simulink model "aero_guidance_train_2026"  (R2026a)
settings: Solver=FixedStepAuto  StopTime=20  FixedStep=0.001  AbsTol=1e-6
PreLoadFcn:
  | aero_guid_dat
StopFcn:
  | %aero_guid_plot
values from neighbouring files (symbols this model uses):
  alpha_vec = (-20:1:20)'*d2r    [aero_guid_dat.m]
  Beamwidth = 10*d2r    (= 0.174532925199)    [aero_guid_dat.m]
  Cm_alpha = am*al.^3 + bm*al.*abs(al) - cm*(7-8*M/3).*al    [aero_guid_dat.m]
  Cm_el = -0.206000/d2r    (= -11.8029305797)    [aero_guid_dat.m]
  Cm_q = -1.719    [aero_guid_dat.m]
  Cx_alpha = -0.3*ones(length(alpha_vec),length(Mach_vec))    [aero_guid_dat.m]
  Cz_alpha = an*al.^3 + bn*al.*abs(al) + cn*(2-M/3).*al    [aero_guid_dat.m]
  Cz_el = -0.034000/d2r    (= -1.94805650344)    [aero_guid_dat.m]
  d2r = pi/180    (= 0.0174532925199)    [aero_guid_dat.m]
  d_ref = 0.75/m2ft    (= 0.228599992685)    [aero_guid_dat.m]
  fin_max = 30.0*d2r    (= 0.523598775598)    [aero_guid_dat.m]
  fin_min = -30.0*d2r    (= -0.523598775598)    [aero_guid_dat.m]
  g = 9.81    [aero_guid_dat.m]
  Goal_pos = [4800; -3200]    [aero_guid_dat.m]
  h_ini = 10000/m2ft    (= 3047.99990246)    [aero_guid_dat.m]
  K_r = -0.02    [aero_guid_dat.m]
  Ks = wgyro/5    (= 125.663706144)    [aero_guid_dat.m]
  l_acc = 0.5    [aero_guid_dat.m]
  Mach_vec = 2:0.5:4    [aero_guid_dat.m]
  max_acc = 40*9.81    (= 392.4)    [aero_guid_dat.m]
  max_gimbal = 35*d2r    (= 0.610865238198)    [aero_guid_dat.m]
  min_gimbal = -35*d2r    (= -0.610865238198)    [aero_guid_dat.m]
  q_ini = 0*d2r    (= 0)    [aero_guid_dat.m]
  R_scale = 5000    [aero_guid_dat.m]
  S_ref = 0.44/m2ft^2    (= 0.0408773349839)    [aero_guid_dat.m]
  target_dt = 0.01    [aero_guid_dat.m]
  target_init_pos = pos_tgt(:)    [aero_guid_dat.m]
  target_max_turn_rate = 120 * (pi/180)    (= 2.09439510239)    [aero_guid_dat.m]
  theta_tgt = 180*d2r    (= 3.14159265359)    [aero_guid_dat.m]
  Thrust = 10e3    (= 10000)    [aero_guid_dat.m]
  tors = 0.05    [aero_guid_dat.m]
  v_ini = 3*328    (= 984)    [aero_guid_dat.m]
  V_scale = 1000    [aero_guid_dat.m]
  v_tgt = 328    [aero_guid_dat.m]
  wgyro = 100*2*pi    (= 628.318530718)    [aero_guid_dat.m]
  wn_hom = 7.0    (= 7)    [aero_guid_dat.m]
  x_ini = 0    [aero_guid_dat.m]
undefined symbols (not defined in the file or in its folder): alpha_sch, K, Ka, Kg, Ki, M_sch
libraries: aerolibasang x3, simulink x2, aerolibanim x1, aerolibatmos2 x1, aerolibactuator x1, rllib x1
CloseFcn:
  | h=findobj('type','figure');if ~isempty(h);close(h);end
Description:
  | Dynamics of a missile engaging a target which is flying straight and level
settings Model: ExtModeTrigMode=oneshot  ExtModeArmWhenConnect=off  ExtModeAutoUpdateStatusClock=off  Creator=The MathWorks, Inc.  LastModifiedBy=yunho
settings DataIOCC: StateSaveName=xbase  OutputSaveName=ybase  SignalLoggingName=sigsOut
settings OptimizationCC: InitFltsAndDblsToZero=on
settings DebuggingCC: SaveWithParameterizedLinksMsg=none  SignalResolutionControl=TryResolveAllWithWarning  MultiTaskDSMMsg=warning  MultiTaskCondExecSysMsg=none  SigSpecEnsureSampleTimeMsg=none
settings HardwareCC: ProdHWDeviceType=32-bit Generic
settings GRTTargetCC: TargetFcnLib=ansi_tfl_tmw.mat  CombineOutputUpdateFcns=off  GRTInterface=on
settings ConfigComp: CovMetricSettings=d

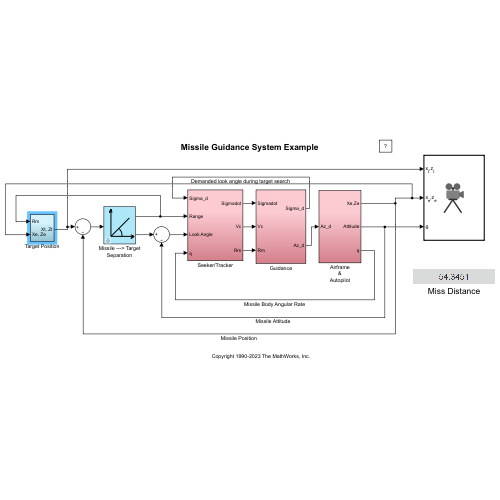
[thumbnail: Simulink's stored preview of the top-level diagram]
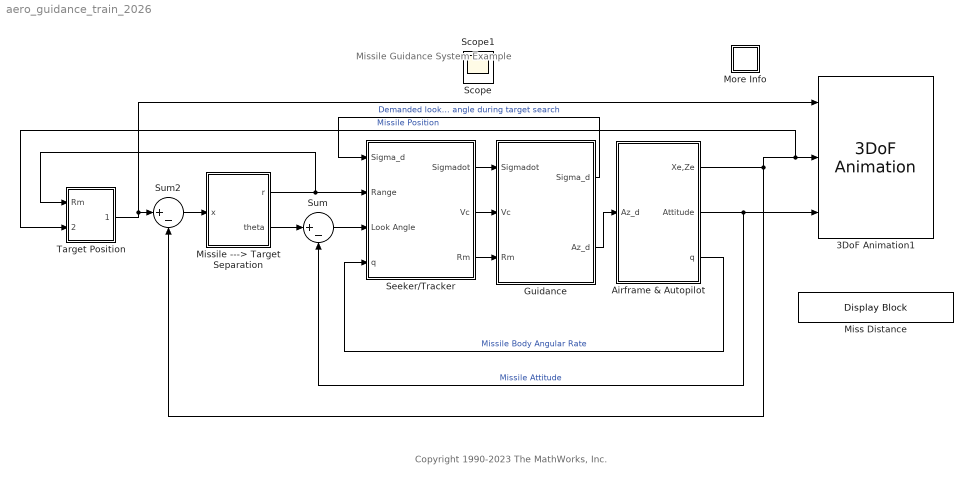
== system aero_guidance_train_2026 ==
  note: Copyright 1990-2023 The MathWorks, Inc.
  note: Missile Guidance System Example
  3DoF Animation1 : aerolibanim/3DoF Animation  u1=[0 5000 -2000 2000 -5050 -3050]  u2=0.01  u3=4  u5=Fixed position  u6=[2500 4000 -4050]  u7=40  u8=on
  Airframe & Autopilot : Subsystem
  Guidance : Subsystem
  Miss Distance : DisplayBlock  LabelPosition=Hide  Transparency=1  GridColor=[0.0, 0.0, 0.0]
  Missile ---> Target Separation : Subsystem  mask(Cart2Polar){}
      mask help:
      | Transformation from cartesian to polar coordinates.
      | [x, y] -> [r, theta]
      |
      | r = sqrt(x^2 + y^2);
      | theta = atan(y/x);
      mask Help: Unmask this block for more help.
      mask Display: plot(0,0,100,100,[24,20,15,20,20],[85,95,85,95,20],[80,20,95,85,95,85],[70,20,20,15,20,24],[56,56,55,52,50,46],[20,26,31,35,38,42])
  More Info : Subsystem
      settings: OpenFcn=showExample('simulink_aerospace/DesigningAGuidanceSystemInMATLABAndSimulinkExample')
      mask Display: disp('?')
  Seeker/Tracker : Subsystem
  Sum : Sum  Inputs=|+-  InputSameDT=on  SaturateOnIntegerOverflow=on  OutDataTypeStr=Inherit: Same as first input
  Sum2 : Sum  Inputs=|+-  InputSameDT=on  SaturateOnIntegerOverflow=on  OutDataTypeStr=Inherit: Same as first input
  Target Position : Subsystem
  Scope : Scope
  Scope1 : Scope
  wires:
  Missile ---> Target Separation/2(theta) -> Sum/1
  Guidance/2(Az_d) -> Airframe & Autopilot/1(Az_d)
  Seeker/Tracker/2(Vc) -> Guidance/2(Vc)
  Seeker/Tracker/3(Rm) -> Guidance/3(Rm)
  Seeker/Tracker/1(Sigmadot) -> Guidance/1(Sigmadot)
  Sum/1 -> Seeker/Tracker/3(Look Angle)
  Airframe & Autopilot/3(q) -> Seeker/Tracker/4(q)  "Missile Body Angular Rate"
  Guidance/1(Sigma_d) -> Seeker/Tracker/1(Sigma_d)  "Demanded look angle during target search"
  Missile ---> Target Separation/1(r) -> Target Position/1(Rm), Seeker/Tracker/2(Range)
  Airframe & Autopilot/1(Xe,Ze) -> Target Position/2("Xe, Ze"), 3DoF Animation1/2, Sum2/2  "Missile Position"
  Airframe & Autopilot/2(Attitude) -> Sum/2, 3DoF Animation1/3  "Missile Attitude"
  Sum2/1 -> Missile ---> Target Separation/1(x)
  Target Position/1("Xt, Zt") -> 3DoF Animation1/1, Sum2/1

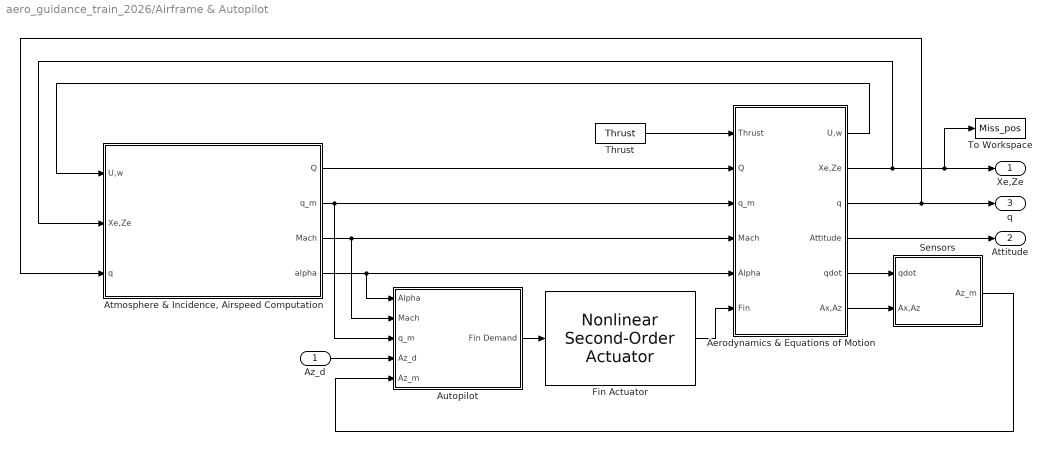
== system aero_guidance_train_2026/Airframe & Autopilot ==
  Az_d : Inport
  Aerodynamics & Equations of Motion : Subsystem
  "Atmosphere & Incidence, Airspeed Computation" : Subsystem
  Autopilot : Subsystem
  Fin Actuator : aerolibactuator/Nonlinear Second-Order Actuator  wn_fin=wn_fin  z_fin=z_fin  fin_max=fin_max  fin_min=fin_min  fin_maxrate=fin_maxrate  fin_act_0=fin_act_0  fin_act_vel=0
  Sensors : Subsystem
  Thrust : Constant  Value=Thrust
  To Workspace : ToWorkspace  VariableName=Miss_pos  SaveFormat=Structure With Time  SampleTime=-1
  Xe,Ze : Outport  InitialOutput=0  VectorParamsAs1DForOutWhenUnconnected=off
  Attitude : Outport  Port=2  InitialOutput=0  VectorParamsAs1DForOutWhenUnconnected=off
  q : Outport  Port=3  InitialOutput=0  VectorParamsAs1DForOutWhenUnconnected=off
  wires:
  Thrust/1 -> Aerodynamics & Equations of Motion/1(Thrust)
  Aerodynamics & Equations of Motion/3(q) -> q/1, "Atmosphere & Incidence, Airspeed Computation"/3(q)
  Aerodynamics & Equations of Motion/2(Xe,Ze) -> To Workspace/1, Xe,Ze/1, "Atmosphere & Incidence, Airspeed Computation"/2(Xe,Ze)
  "Atmosphere & Incidence, Airspeed Computation"/3(Mach) -> Aerodynamics & Equations of Motion/4(Mach), Autopilot/2(Mach)
  Aerodynamics & Equations of Motion/1(U,w) -> "Atmosphere & Incidence, Airspeed Computation"/1(U,w)
  "Atmosphere & Incidence, Airspeed Computation"/1(Q) -> Aerodynamics & Equations of Motion/2(Q)
  "Atmosphere & Incidence, Airspeed Computation"/4(alpha) -> Autopilot/1(Alpha), Aerodynamics & Equations of Motion/5(Alpha)
  "Atmosphere & Incidence, Airspeed Computation"/2(q_m) -> Aerodynamics & Equations of Motion/3(q_m), Autopilot/3(q_m)
  Aerodynamics & Equations of Motion/4(Attitude) -> Attitude/1
  Aerodynamics & Equations of Motion/5(qdot) -> Sensors/1(qdot)
  Aerodynamics & Equations of Motion/6(Ax,Az) -> Sensors/2(Ax,Az)
  Autopilot/1(Fin Demand) -> Fin Actuator/1
  Fin Actuator/1 -> Aerodynamics & Equations of Motion/6(Fin)
  Az_d/1 -> Autopilot/4(Az_d)
  Sensors/1(Az_m) -> Autopilot/5(Az_m)

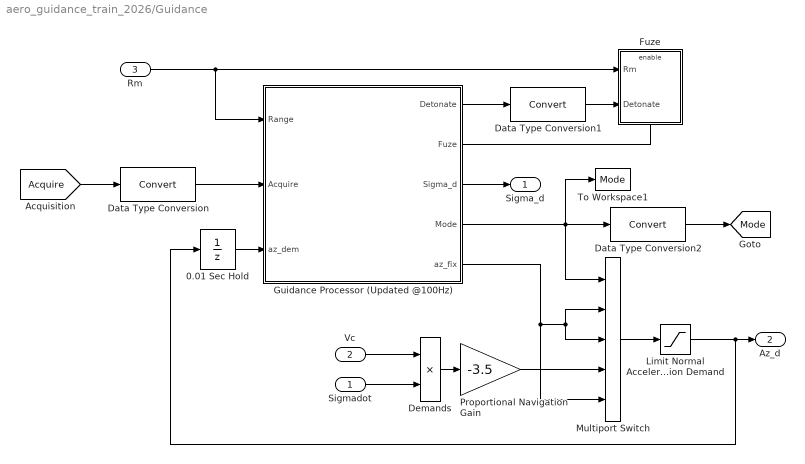
== system aero_guidance_train_2026/Guidance ==
  Sigmadot : Inport
  Vc : Inport  Port=2
  Rm : Inport  Port=3
  0.01 Sec Hold : UnitDelay  SampleTime=0.01
  Data Type Conversion : DataTypeConversion  SaturateOnIntegerOverflow=off  RndMeth=Floor
  Data Type Conversion1 : DataTypeConversion  SaturateOnIntegerOverflow=off  RndMeth=Floor
  Data Type Conversion2 : DataTypeConversion  SaturateOnIntegerOverflow=off  RndMeth=Floor
  Demands : Product  InputSameDT=on  SaturateOnIntegerOverflow=on  OutDataTypeStr=Inherit: Same as first input
  Fuze : Subsystem  TreatAsAtomicUnit=on
  Guidance Processor (Updated @100Hz) : Stateflow chart  TreatAsAtomicUnit=on
  "Limit Normal Acceleration Demand " : Saturate  UpperLimit=max_acc  LowerLimit=-max_acc
  Multiport Switch : MultiPortSwitch  Inputs=4
  Proportional Navigation Gain : Gain  Gain=-3.5  SaturateOnIntegerOverflow=on  OutDataTypeStr=Inherit: Same as input  ParamDataTypeStr=Inherit: Same as input
  To Workspace1 : ToWorkspace  VariableName=Mode  SaveFormat=Structure With Time
  Sigma_d : Outport  VectorParamsAs1DForOutWhenUnconnected=off
  Az_d : Outport  Port=2  VectorParamsAs1DForOutWhenUnconnected=off
  tag scope: Mode=global
  wires:
  Guidance Processor (Updated @100Hz)/3(Sigma_d) -> Sigma_d/1
  [Acquire] -> Data Type Conversion/1
  Multiport Switch/1 -> "Limit Normal Acceleration Demand "/1
  Guidance Processor (Updated @100Hz)/1(Detonate) -> Data Type Conversion1/1
  "Limit Normal Acceleration Demand "/1 -> Az_d/1, 0.01 Sec Hold/1
  Guidance Processor (Updated @100Hz)/5(az_fix) -> Multiport Switch/2, Multiport Switch/3, Multiport Switch/5
  0.01 Sec Hold/1 -> Guidance Processor (Updated @100Hz)/3(az_dem)
  Sigmadot/1 -> Demands/2
  Proportional Navigation Gain/1 -> Multiport Switch/4
  Vc/1 -> Demands/1
  Demands/1 -> Proportional Navigation Gain/1
  Rm/1 -> Fuze/1(Rm), Guidance Processor (Updated @100Hz)/1(Range)
  Guidance Processor (Updated @100Hz)/2(Fuze) -> Fuze/Enable
  Guidance Processor (Updated @100Hz)/4(Mode) -> Data Type Conversion2/1, To Workspace1/1, Multiport Switch/1
  Data Type Conversion/1 -> Guidance Processor (Updated @100Hz)/2(Acquire)
  Data Type Conversion1/1 -> Fuze/2(Detonate)
  Data Type Conversion2/1 -> [Mode]

== system aero_guidance_train_2026/Missile ---> Target Separation ==
  x : Inport
  Range : Fcn  Expr=hypot(u[1],u[2])
  Sightline Angle : Fcn  Expr=atan2(-u[2],u[1])
  r : Outport  InitialOutput=0  VectorParamsAs1DForOutWhenUnconnected=off
  theta : Outport  Port=2  InitialOutput=0  VectorParamsAs1DForOutWhenUnconnected=off
  wires:
  x/1 -> Sightline Angle/1, Range/1
  Range/1 -> r/1
  Sightline Angle/1 -> theta/1

== system aero_guidance_train_2026/More Info ==

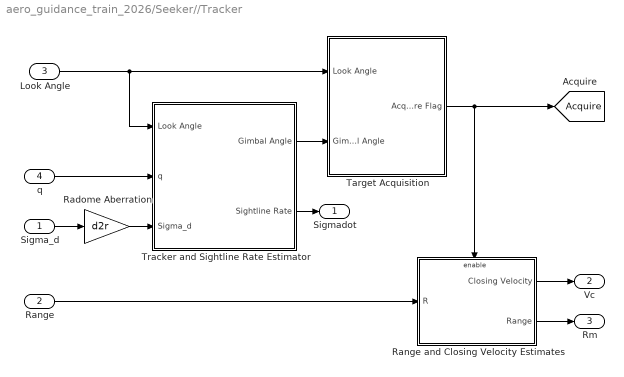
== system aero_guidance_train_2026/Seeker//Tracker ==
  Sigma_d : Inport
  Range : Inport  Port=2
  Look Angle : Inport  Port=3
  q : Inport  Port=4
  Radome Aberration : Gain  Gain=d2r  SaturateOnIntegerOverflow=on  OutDataTypeStr=Inherit: Same as input  ParamDataTypeStr=Inherit: Same as input
  Range and Closing Velocity Estimates : Subsystem  TreatAsAtomicUnit=on
  Target Acquisition : Subsystem
  Tracker and Sightline Rate Estimator : Subsystem
  Sigmadot : Outport  VectorParamsAs1DForOutWhenUnconnected=off
  Vc : Outport  Port=2  VectorParamsAs1DForOutWhenUnconnected=off
  Rm : Outport  Port=3  VectorParamsAs1DForOutWhenUnconnected=off
  tag scope: Acquire=global
  wires:
  Tracker and Sightline Rate Estimator/2(Sightline Rate) -> Sigmadot/1
  Radome Aberration/1 -> Tracker and Sightline Rate Estimator/3(Sigma_d)
  Tracker and Sightline Rate Estimator/1("Gimbal Angle ") -> Target Acquisition/2(Gimbal Angle)
  Target Acquisition/1(Acquire Flag) -> [Acquire], Range and Closing Velocity Estimates/Enable
  q/1 -> Tracker and Sightline Rate Estimator/2(q)
  Look Angle/1 -> Target Acquisition/1(Look Angle), Tracker and Sightline Rate Estimator/1(Look Angle)
  Range/1 -> Range and Closing Velocity Estimates/1(R)
  Range and Closing Velocity Estimates/2(Range) -> Rm/1
  Range and Closing Velocity Estimates/1(Closing Velocity) -> Vc/1
  Sigma_d/1 -> Radome Aberration/1

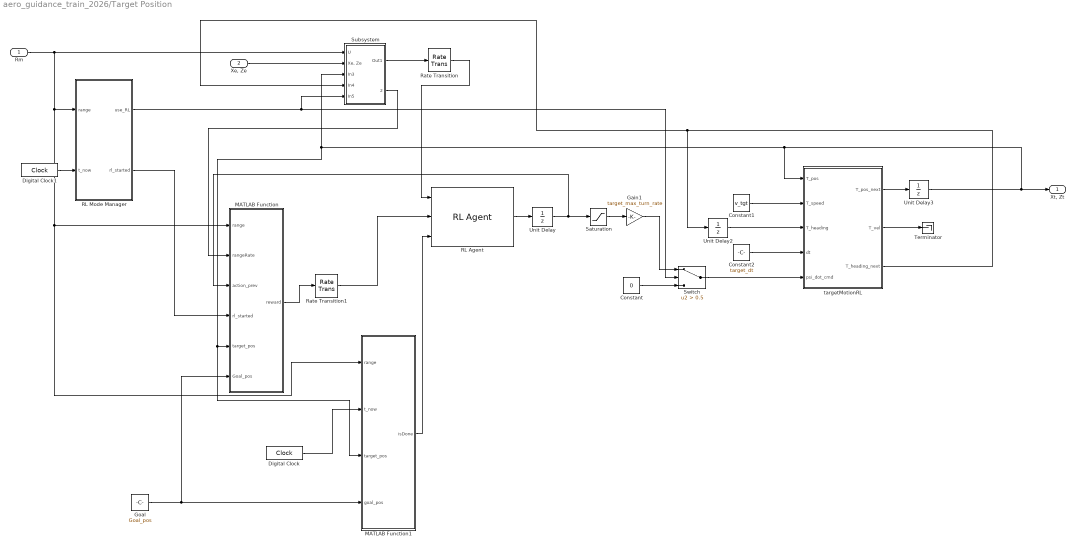
== system aero_guidance_train_2026/Target Position ==
  Rm : Inport
  "Xe, Ze" : Inport  Port=2
  Constant : Constant  Value=0
  Constant1 : Constant  Value=v_tgt
  Constant2 : Constant  Value=target_dt
  Digital Clock : DigitalClock  SampleTime=target_dt
  Digital Clock1 : DigitalClock  SampleTime=target_dt
  Gain1 : Gain  Gain=target_max_turn_rate
  Goal : Constant  Value=Goal_pos  SampleTime=target_dt
  MATLAB Function : MATLAB Function  TreatAsAtomicUnit=on
  MATLAB Function1 : MATLAB Function  TreatAsAtomicUnit=on
  RL Agent : rllib/RL Agent  Agent=agent  ExternalActionAsInput=off  ProvideLastAction=off  ProvideCumRwd=off  TreatAsDirectFeedthrough=on  UseStrictObservationDataTypes=off
  RL Mode Manager : MATLAB Function  TreatAsAtomicUnit=on  SystemSampleTime=target_dt
  Rate Transition : RateTransition  OutPortSampleTime=target_dt
  Rate Transition1 : RateTransition  OutPortSampleTime=target_dt
  Saturation : Saturate  UpperLimit=1  LowerLimit=-1
  Subsystem : Subsystem
  Switch : Switch  Criteria=u2 > Threshold  Threshold=0.5  SaturateOnIntegerOverflow=off  InputSameDT=off
  Terminator : Terminator
  Unit Delay : UnitDelay  SampleTime=0.01
  Unit Delay2 : UnitDelay  InitialCondition=theta_tgt  SampleTime=target_dt
  Unit Delay3 : UnitDelay  InitialCondition=target_init_pos  SampleTime=target_dt
  targetMotionRL : MATLAB Function  TreatAsAtomicUnit=on  SystemSampleTime=target_dt
  "Xt, Zt" : Outport
  wires:
  RL Agent/1 -> Unit Delay/1
  Saturation/1 -> Gain1/1
  Gain1/1 -> Switch/1
  RL Mode Manager/1(use_RL) -> Subsystem/5(In5), Switch/2
  Constant/1 -> Switch/3
  Switch/1 -> targetMotionRL/5(psi_dot_cmd)
  Rm/1 -> MATLAB Function1/1(range), MATLAB Function/1(range), RL Mode Manager/1(range), Subsystem/1(U)
  "Xe, Ze"/1 -> Subsystem/2("Xe, Ze")
  targetMotionRL/1(T_pos_next) -> Unit Delay3/1
  targetMotionRL/3(T_heading_next) -> Subsystem/4(In4), Unit Delay2/1
  Subsystem/2(rangeRate_raw) -> MATLAB Function/2(rangeRate)
  Unit Delay/1 -> Saturation/1, MATLAB Function/3(action_prev)
  RL Mode Manager/2(rl_started) -> MATLAB Function/4(rl_started)
  Digital Clock/1 -> MATLAB Function1/2(t_now)
  Constant1/1 -> targetMotionRL/2(T_speed)
  Unit Delay2/1 -> targetMotionRL/3(T_heading)
  Constant2/1 -> targetMotionRL/4(dt)
  targetMotionRL/2(T_vel) -> Terminator/1
  Subsystem/1(Out1) -> Rate Transition/1
  Rate Transition/1 -> RL Agent/1
  MATLAB Function/1(reward) -> Rate Transition1/1
  Rate Transition1/1 -> RL Agent/2
  Unit Delay3/1 -> targetMotionRL/1(T_pos), MATLAB Function1/3(target_pos), MATLAB Function/5(target_pos), Subsystem/3(In3), "Xt, Zt"/1
  Digital Clock1/1 -> RL Mode Manager/2(t_now)
  MATLAB Function1/1(isDone) -> RL Agent/3
  Goal/1 -> MATLAB Function/6(Goal_pos), MATLAB Function1/4(goal_pos)

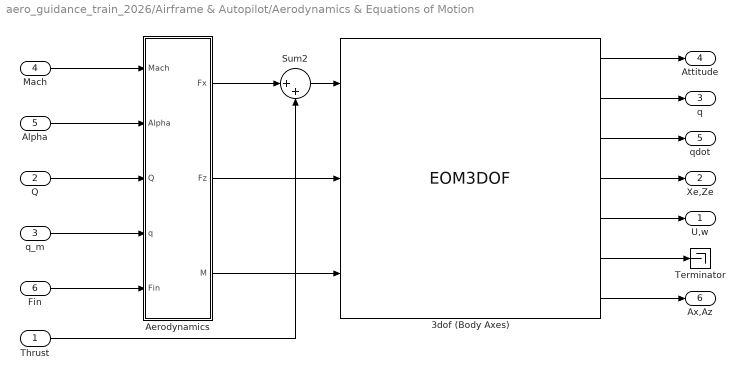
== system aero_guidance_train_2026/Airframe & Autopilot/Aerodynamics & Equations of Motion ==
  Thrust : Inport
  Q : Inport  Port=2
  q_m : Inport  Port=3
  Mach : Inport  Port=4
  Alpha : Inport  Port=5
  Fin : Inport  Port=6
  3dof (Body Axes) : EOM3DOF  v_ini=v_ini  theta_ini=theta_ini  q_ini=q_ini  alpha_ini=alpha_ini  pos_ini=[x_ini -h_ini]  mass=mass  Iyy=Iyy  g=g  abi_flag=on
  Aerodynamics : Subsystem
  Sum2 : Sum  Inputs=|++  InputSameDT=on  SaturateOnIntegerOverflow=on  OutDataTypeStr=Inherit: Same as first input
  Terminator : Terminator
  U,w : Outport  InitialOutput=0  VectorParamsAs1DForOutWhenUnconnected=off
  Xe,Ze : Outport  Port=2  InitialOutput=0  VectorParamsAs1DForOutWhenUnconnected=off
  q : Outport  Port=3  InitialOutput=0  VectorParamsAs1DForOutWhenUnconnected=off
  Attitude : Outport  Port=4  InitialOutput=0  VectorParamsAs1DForOutWhenUnconnected=off
  qdot : Outport  Port=5  InitialOutput=0  VectorParamsAs1DForOutWhenUnconnected=off
  Ax,Az : Outport  Port=6  InitialOutput=0  VectorParamsAs1DForOutWhenUnconnected=off
  wires:
  Aerodynamics/3(" M") -> 3dof (Body Axes)/3
  Sum2/1 -> 3dof (Body Axes)/1
  Fin/1 -> Aerodynamics/5(Fin)
  Aerodynamics/2(Fz) -> 3dof (Body Axes)/2
  Aerodynamics/1(Fx) -> Sum2/1
  Thrust/1 -> Sum2/2
  q_m/1 -> Aerodynamics/4(q)
  Mach/1 -> Aerodynamics/1(Mach)
  Q/1 -> Aerodynamics/3(Q)
  Alpha/1 -> Aerodynamics/2(Alpha)
  3dof (Body Axes)/7 -> Ax,Az/1
  3dof (Body Axes)/6 -> Terminator/1
  3dof (Body Axes)/5 -> U,w/1
  3dof (Body Axes)/4 -> Xe,Ze/1
  3dof (Body Axes)/3 -> qdot/1
  3dof (Body Axes)/2 -> q/1
  3dof (Body Axes)/1 -> Attitude/1

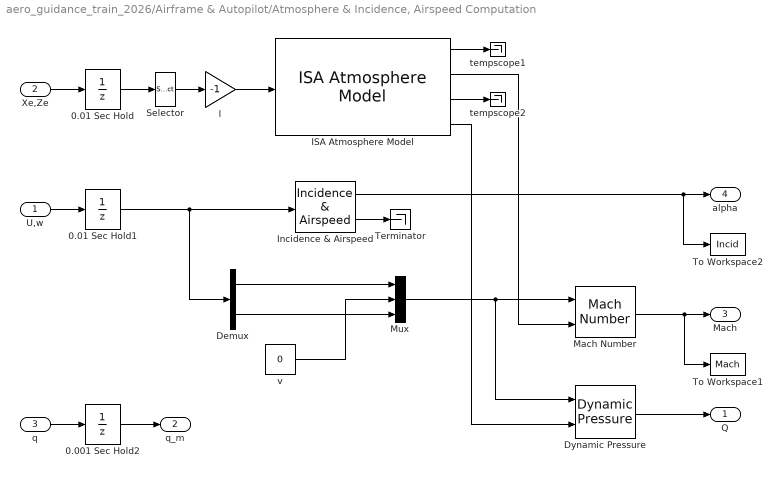
== system aero_guidance_train_2026/Airframe & Autopilot/Atmosphere & Incidence, Airspeed Computation ==
  U,w : Inport
  Xe,Ze : Inport  Port=2
  q : Inport  Port=3
  0.001 Sec Hold2 : UnitDelay  InitialCondition=q_ini  SampleTime=0.001
  0.01 Sec Hold : UnitDelay  InitialCondition=[x_ini -h_ini]  SampleTime=0.01
  0.01 Sec Hold1 : UnitDelay  InitialCondition=[v_ini 0]  SampleTime=0.01
  Demux : Demux  Outputs=2
  Dynamic Pressure : aerolibasang/Dynamic Pressure
  ISA Atmosphere Model : aerolibatmos2/ISA Atmosphere Model  useExtended=off  action=Warning  custom=off  viscosityOut=off  g=9.80665  gamma=1.4  R=287.0531  L=0.0065  h_trop=11000  h_strat=20000  rho0=1.225  P0=101325  T0=288.15  h0=0  S=110.4  Tref=273.15  muref=1.716e-5
  Incidence & Airspeed : aerolibasang/Incidence  & Airspeed
  Mach Number : aerolibasang/Mach Number
  Mux : Mux  Inputs=3
  Selector : Selector  InputPortWidth=2  IndexOptions=Index vector (dialog)  Indices=[2]  OutputSizes=1
  Terminator : Terminator
  To Workspace1 : ToWorkspace  VariableName=Mach  SaveFormat=Structure With Time  SampleTime=-1
  To Workspace2 : ToWorkspace  VariableName=Incid  SaveFormat=Structure With Time  SampleTime=-1
  l : Gain  Gain=-1  SaturateOnIntegerOverflow=on  OutDataTypeStr=Inherit: Same as input  ParamDataTypeStr=Inherit: Same as input
  tempscope1 : Terminator
  tempscope2 : Terminator
  v : Constant  Value=0
  Q : Outport
  q_m : Outport  Port=2
  Mach : Outport  Port=3
  alpha : Outport  Port=4
  wires:
  U,w/1 -> 0.01 Sec Hold1/1
  Incidence & Airspeed/1 -> To Workspace2/1, alpha/1
  Demux/1 -> Mux/1
  Demux/2 -> Mux/3
  v/1 -> Mux/2
  Mux/1 -> Mach Number/1, Dynamic Pressure/1
  Incidence & Airspeed/2 -> Terminator/1
  ISA Atmosphere Model/4 -> Dynamic Pressure/2
  Mach Number/1 -> To Workspace1/1, Mach/1
  Dynamic Pressure/1 -> Q/1
  0.01 Sec Hold1/1 -> Incidence & Airspeed/1, Demux/1
  0.01 Sec Hold/1 -> Selector/1
  l/1 -> ISA Atmosphere Model/1
  ISA Atmosphere Model/1 -> tempscope1/1
  ISA Atmosphere Model/3 -> tempscope2/1
  Selector/1 -> l/1
  Xe,Ze/1 -> 0.01 Sec Hold/1
  ISA Atmosphere Model/2 -> Mach Number/2
  0.001 Sec Hold2/1 -> q_m/1
  q/1 -> 0.001 Sec Hold2/1

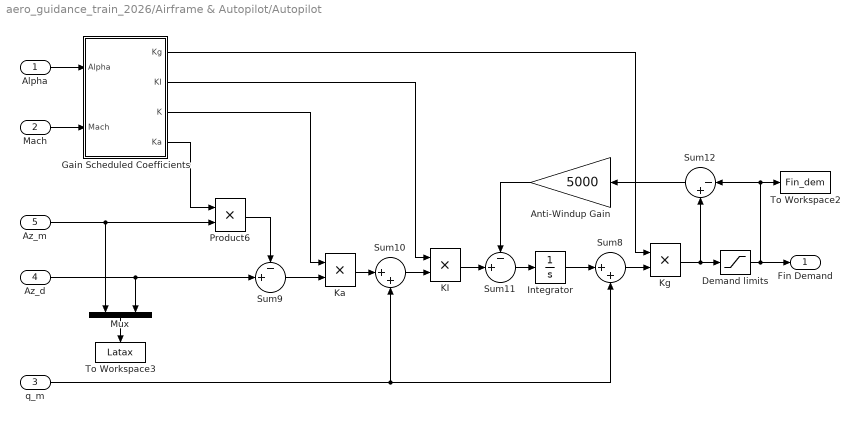
== system aero_guidance_train_2026/Airframe & Autopilot/Autopilot ==
  Alpha : Inport
  Mach : Inport  Port=2
  q_m : Inport  Port=3
  Az_d : Inport  Port=4
  Az_m : Inport  Port=5
  Anti-Windup Gain : Gain  Gain=5000  SaturateOnIntegerOverflow=on  OutDataTypeStr=Inherit: Same as input  ParamDataTypeStr=Inherit: Same as input
  "Demand limits " : Saturate  UpperLimit=fin_max  LowerLimit=fin_min
  Gain Scheduled Coefficients : Subsystem
  Integrator : Integrator
  KI : Product  InputSameDT=on  SaturateOnIntegerOverflow=on  OutDataTypeStr=Inherit: Same as first input
  Ka : Product  InputSameDT=on  SaturateOnIntegerOverflow=on  OutDataTypeStr=Inherit: Same as first input
  Kg : Product  InputSameDT=on  SaturateOnIntegerOverflow=on  OutDataTypeStr=Inherit: Same as first input
  Mux : Mux  Inputs=2
  Product6 : Product  InputSameDT=on  SaturateOnIntegerOverflow=on  OutDataTypeStr=Inherit: Same as first input
  Sum10 : Sum  Inputs=|++  InputSameDT=on  SaturateOnIntegerOverflow=on  OutDataTypeStr=Inherit: Same as first input
  Sum11 : Sum  Inputs=-+|  InputSameDT=on  SaturateOnIntegerOverflow=on  OutDataTypeStr=Inherit: Same as first input
  Sum12 : Sum  Inputs=|-+  InputSameDT=on  SaturateOnIntegerOverflow=on  OutDataTypeStr=Inherit: Same as first input
  Sum8 : Sum  Inputs=|++  InputSameDT=on  SaturateOnIntegerOverflow=on  OutDataTypeStr=Inherit: Same as first input
  Sum9 : Sum  Inputs=-+|  InputSameDT=on  SaturateOnIntegerOverflow=on  OutDataTypeStr=Inherit: Same as first input
  To Workspace2 : ToWorkspace  VariableName=Fin_dem  SaveFormat=Structure With Time  SampleTime=-1
  To Workspace3 : ToWorkspace  VariableName=Latax  SaveFormat=Structure With Time  SampleTime=-1
  Fin Demand : Outport  InitialOutput=0  VectorParamsAs1DForOutWhenUnconnected=off
  wires:
  Mach/1 -> Gain Scheduled Coefficients/2(Mach)
  Alpha/1 -> Gain Scheduled Coefficients/1(Alpha)
  Kg/1 -> Sum12/2, "Demand limits "/1
  Gain Scheduled Coefficients/1("Kg ") -> Kg/1
  Gain Scheduled Coefficients/3("K ") -> Ka/1
  Gain Scheduled Coefficients/2("KI ") -> KI/1
  Anti-Windup Gain/1 -> Sum11/1
  Sum8/1 -> Kg/2
  Integrator/1 -> Sum8/1
  Sum11/1 -> Integrator/1
  Product6/1 -> Sum9/1
  Sum9/1 -> Ka/2
  Ka/1 -> Sum10/1
  Sum10/1 -> KI/2
  KI/1 -> Sum11/2
  Sum12/1 -> Anti-Windup Gain/1
  Az_d/1 -> Mux/2, Sum9/2
  Mux/1 -> To Workspace3/1
  q_m/1 -> Sum10/2, Sum8/2
  "Demand limits "/1 -> Fin Demand/1, Sum12/1, To Workspace2/1
  Az_m/1 -> Mux/1, Product6/2
  Gain Scheduled Coefficients/4("Ka ") -> Product6/1

== system aero_guidance_train_2026/Airframe & Autopilot/Sensors ==
  qdot : Inport
  Ax,Az : Inport  Port=2
  Selector : Selector  InputPortWidth=2  IndexOptions=Index vector (dialog)  Indices=[2]  OutputSizes=1
  Sum : Sum  Inputs=-+|  InputSameDT=on  SaturateOnIntegerOverflow=on  OutDataTypeStr=Inherit: Same as first input
  l : Gain  Gain=l_acc  SaturateOnIntegerOverflow=on  OutDataTypeStr=Inherit: Same as input  ParamDataTypeStr=Inherit: Same as input
  Az_m : Outport  InitialOutput=0  VectorParamsAs1DForOutWhenUnconnected=off
  wires:
  Selector/1 -> Sum/2
  Ax,Az/1 -> Selector/1
  l/1 -> Sum/1
  Sum/1 -> Az_m/1  "Accelerometer"
  qdot/1 -> l/1

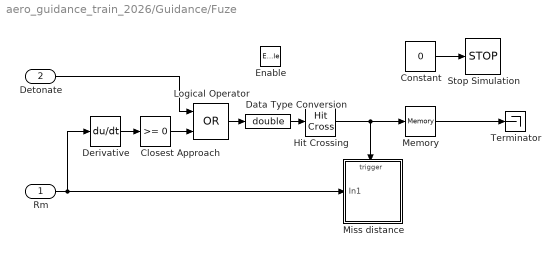
== system aero_guidance_train_2026/Guidance/Fuze ==
  Rm : Inport
  Detonate : Inport  Port=2
  Enable : EnablePort
  Closest Approach : simulink/Logic and Bit Operations/Compare To Zero  relop=>=  OutDataTypeStr=boolean
  Constant : Constant  Value=0
  Data Type Conversion : DataTypeConversion  OutDataTypeStr=double  SaturateOnIntegerOverflow=off  RndMeth=Floor
  Derivative : Derivative
  Hit Crossing : HitCross  HitCrossingDirection=rising
  Logical Operator : Logic  Operator=OR  IconShape=distinctive  OutDataTypeStr=boolean
  Memory : Memory
  Miss distance : Subsystem  TreatAsAtomicUnit=on
  Stop Simulation : Stop
  Terminator : Terminator
  wires:
  Derivative/1 -> Closest Approach/1
  Detonate/1 -> Logical Operator/1
  Rm/1 -> Miss distance/1(In1), Derivative/1
  Closest Approach/1 -> Logical Operator/2
  Memory/1 -> Terminator/1
  Hit Crossing/1 -> Miss distance/Trigger, Memory/1
  Data Type Conversion/1 -> Hit Crossing/1
  Logical Operator/1 -> Data Type Conversion/1
  Constant/1 -> Stop Simulation/1

== system aero_guidance_train_2026/Seeker//Tracker/Range and Closing Velocity Estimates ==
  R : Inport
  Enable : EnablePort  StatesWhenEnabling=reset
  Bandwidth of Estimator : Gain  Gain=wn_hom  SaturateOnIntegerOverflow=on  OutDataTypeStr=Inherit: Same as input  ParamDataTypeStr=Inherit: Same as input
  Initialized at acquisition : Integrator  InitialConditionSource=external
  Rdot ---> Vc : Gain  Gain=-1  SaturateOnIntegerOverflow=on  OutDataTypeStr=Inherit: Same as input  ParamDataTypeStr=Inherit: Same as input
  Sum : Sum  Inputs=|+-  InputSameDT=on  SaturateOnIntegerOverflow=on  OutDataTypeStr=Inherit: Same as first input
  Closing Velocity : Outport  InitialOutput=0  VectorParamsAs1DForOutWhenUnconnected=off
  Range : Outport  Port=2  InitialOutput=0  VectorParamsAs1DForOutWhenUnconnected=off
  wires:
  R/1 -> Range/1, Initialized at acquisition/2, Sum/1
  Sum/1 -> Bandwidth of Estimator/1
  Initialized at acquisition/1 -> Sum/2
  Bandwidth of Estimator/1 -> Rdot ---> Vc/1, Initialized at acquisition/1
  Rdot ---> Vc/1 -> Closing Velocity/1

== system aero_guidance_train_2026/Seeker//Tracker/Target Acquisition ==
  Look Angle : Inport
  Gimbal Angle : Inport  Port=2
  Abs : Abs
  Beamwidth : Constant  Value=Beamwidth/2
  Mux : Mux  Inputs=2
  Relational Operator : RelationalOperator  Operator=<  OutDataTypeStr=boolean
  Sum : Sum  Inputs=+-  InputSameDT=on  SaturateOnIntegerOverflow=on  OutDataTypeStr=Inherit: Same as first input
  To Workspace2 : ToWorkspace  VariableName=Gimbal  SaveFormat=Structure With Time  SampleTime=-1
  Acquire Flag : Outport  VectorParamsAs1DForOutWhenUnconnected=off
  wires:
  Look Angle/1 -> Sum/2, Mux/2
  Gimbal Angle/1 -> Sum/1, Mux/1
  Mux/1 -> To Workspace2/1
  Sum/1 -> Abs/1
  Beamwidth/1 -> Relational Operator/2
  Relational Operator/1 -> Acquire Flag/1
  Abs/1 -> Relational Operator/1

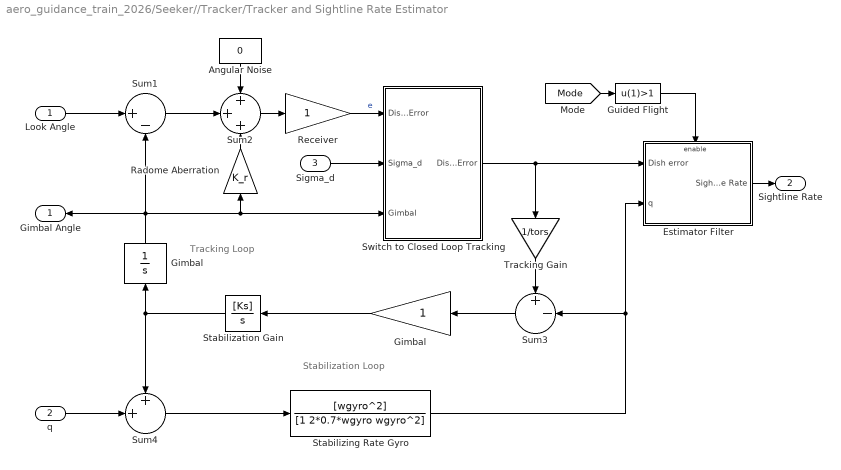
== system aero_guidance_train_2026/Seeker//Tracker/Tracker and Sightline Rate Estimator ==
  note: Stabilization Loop
  note: Tracking Loop
  Look Angle : Inport
  q : Inport  Port=2
  Sigma_d : Inport  Port=3
  Angular Noise : Constant  Value=0
  Estimator Filter : Subsystem  TreatAsAtomicUnit=on
  Gimbal : Gain  SaturateOnIntegerOverflow=on  OutDataTypeStr=Inherit: Same as input  ParamDataTypeStr=Inherit: Same as input
  "Gimbal " : Integrator  LimitOutput=on  UpperSaturationLimit=max_gimbal  LowerSaturationLimit=min_gimbal
  Guided Flight : Fcn  Expr=u(1)>1
  Radome Aberration : Gain  Gain=K_r  SaturateOnIntegerOverflow=on  OutDataTypeStr=Inherit: Same as input  ParamDataTypeStr=Inherit: Same as input
  Receiver : Gain  SaturateOnIntegerOverflow=on  OutDataTypeStr=Inherit: Same as input  ParamDataTypeStr=Inherit: Same as input
  Stabilization Gain : TransferFcn  Numerator=[Ks]  Denominator=[1 0]
  Stabilizing Rate Gyro : TransferFcn  Numerator=[wgyro^2]  Denominator=[1 2*0.7*wgyro wgyro^2]
  Sum1 : Sum  Inputs=|+-  InputSameDT=on  SaturateOnIntegerOverflow=on  OutDataTypeStr=Inherit: Same as first input
  Sum2 : Sum  Inputs=+++  InputSameDT=on  SaturateOnIntegerOverflow=on  OutDataTypeStr=Inherit: Same as first input
  Sum3 : Sum  Inputs=+-|  InputSameDT=on  SaturateOnIntegerOverflow=on  OutDataTypeStr=Inherit: Same as first input
  Sum4 : Sum  Inputs=++|  InputSameDT=on  SaturateOnIntegerOverflow=on  OutDataTypeStr=Inherit: Same as first input
  Switch to Closed Loop Tracking : Subsystem
  Tracking Gain : Gain  Gain=1/tors  SaturateOnIntegerOverflow=on  OutDataTypeStr=Inherit: Same as input  ParamDataTypeStr=Inherit: Same as input
  "Gimbal Angle " : Outport  VectorParamsAs1DForOutWhenUnconnected=off
  Sightline Rate : Outport  Port=2  VectorParamsAs1DForOutWhenUnconnected=off
  wires:
  "Gimbal "/1 -> Sum1/2, Radome Aberration/1, Switch to Closed Loop Tracking/3(Gimbal), "Gimbal Angle "/1
  Stabilization Gain/1 -> "Gimbal "/1, Sum4/1
  Gimbal/1 -> Stabilization Gain/1
  Look Angle/1 -> Sum1/1
  Sum2/1 -> Receiver/1
  Receiver/1 -> Switch to Closed Loop Tracking/1(Dish Error)  "e"
  Sigma_d/1 -> Switch to Closed Loop Tracking/2(Sigma_d)
  Estimator Filter/1(Sightline Rate) -> Sightline Rate/1
  Radome Aberration/1 -> Sum2/3
  Sum1/1 -> Sum2/2
  Angular Noise/1 -> Sum2/1
  Sum4/1 -> Stabilizing Rate Gyro/1
  q/1 -> Sum4/2
  Stabilizing Rate Gyro/1 -> Sum3/2, Estimator Filter/2(q)
  Sum3/1 -> Gimbal/1
  Tracking Gain/1 -> Sum3/1
  Switch to Closed Loop Tracking/1("Dish Error ") -> Tracking Gain/1, Estimator Filter/1(Dish error)
  Guided Flight/1 -> Estimator Filter/Enable
  [Mode] -> Guided Flight/1

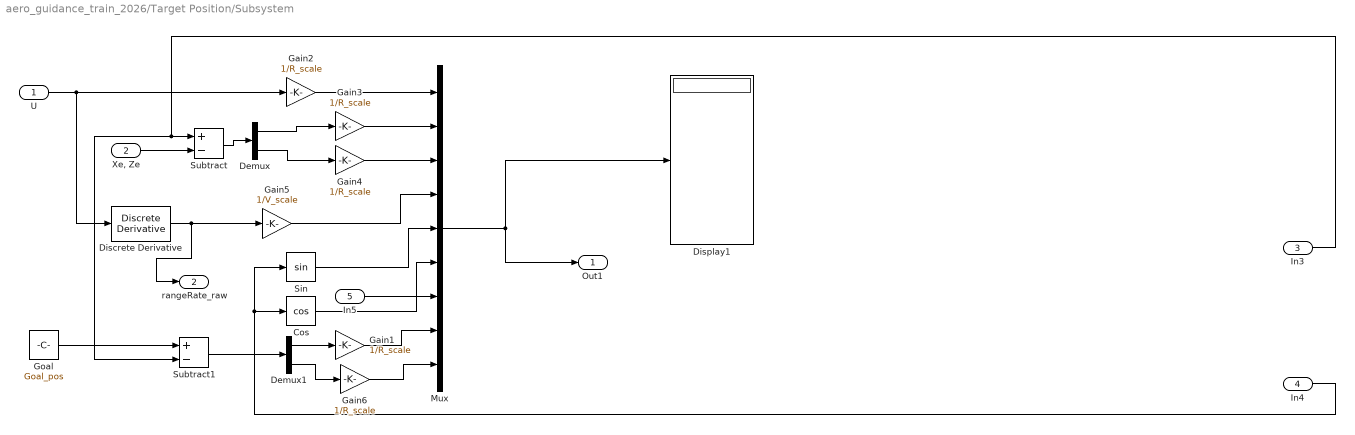
== system aero_guidance_train_2026/Target Position/Subsystem ==
  U : Inport
  "Xe, Ze" : Inport  Port=2
  In3 : Inport  Port=3
  In4 : Inport  Port=4
  In5 : Inport  Port=5
  Cos : Trigonometry  Operator=cos
  Demux : Demux  Outputs=2
  Demux1 : Demux  Outputs=2
  Discrete Derivative : simulink/Discrete/Discrete Derivative  gainval=1.0  ICPrevScaledInput=0.0  OutMin=[]  OutMax=[]  OutDataType=fixdt(1, 16)  OutScaling=2^-10  DoSatur=off
  Display1 : Display
  Gain{1..4,6} (5 alike) : Gain  Gain=1/R_scale
  Gain5 : Gain  Gain=1/V_scale
  Goal : Constant  Value=Goal_pos
  Mux : Mux  Inputs=9
  Sin : Trigonometry
  Subtract : Sum  Inputs=+-
  Subtract1 : Sum  Inputs=+-
  Out1 : Outport
  rangeRate_raw : Outport  Port=2
  wires:
  Demux/2 -> Gain4/1
  U/1 -> Gain2/1, Discrete Derivative/1
  Discrete Derivative/1 -> Gain5/1, rangeRate_raw/1
  Gain5/1 -> Mux/4
  Gain2/1 -> Mux/1
  Gain3/1 -> Mux/2
  Sin/1 -> Mux/5
  Gain4/1 -> Mux/3
  Cos/1 -> Mux/6
  "Xe, Ze"/1 -> Subtract/2
  Subtract/1 -> Demux/1
  Demux/1 -> Gain3/1
  In4/1 -> Cos/1, Sin/1
  Mux/1 -> Out1/1, Display1/1
  In5/1 -> Mux/7
  In3/1 -> Subtract1/2, Subtract/1
  Goal/1 -> Subtract1/1
  Subtract1/1 -> Demux1/1
  Demux1/1 -> Gain1/1
  Demux1/2 -> Gain6/1
  Gain1/1 -> Mux/8
  Gain6/1 -> Mux/9

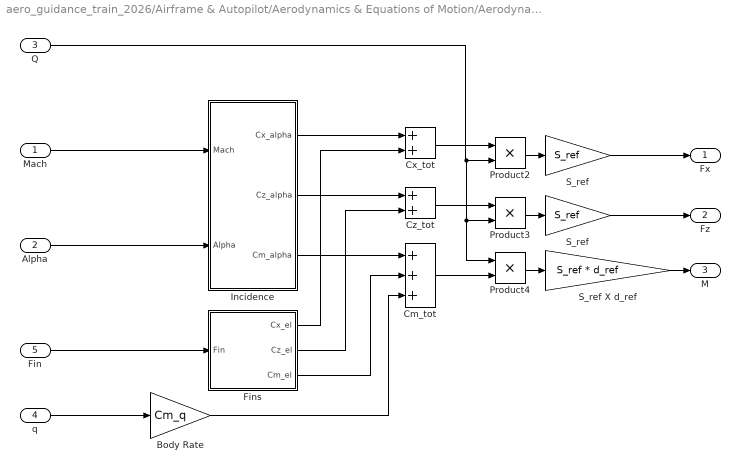
== system aero_guidance_train_2026/Airframe & Autopilot/Aerodynamics & Equations of Motion/Aerodynamics ==
  Mach : Inport
  Alpha : Inport  Port=2
  Q : Inport  Port=3
  q : Inport  Port=4
  Fin : Inport  Port=5
  Body Rate : Gain  Gain=Cm_q  SaturateOnIntegerOverflow=on  OutDataTypeStr=Inherit: Same as input  ParamDataTypeStr=Inherit: Same as input
  Cm_tot : Sum  Inputs=+++  InputSameDT=on  SaturateOnIntegerOverflow=on  OutDataTypeStr=Inherit: Same as first input
  Cx_tot : Sum  InputSameDT=on  SaturateOnIntegerOverflow=on  OutDataTypeStr=Inherit: Same as first input
  Cz_tot : Sum  InputSameDT=on  SaturateOnIntegerOverflow=on  OutDataTypeStr=Inherit: Same as first input
  Fins : Subsystem
  Incidence : Subsystem
  Product2 : Product  InputSameDT=on  SaturateOnIntegerOverflow=on  OutDataTypeStr=Inherit: Same as first input
  Product3 : Product  InputSameDT=on  SaturateOnIntegerOverflow=on  OutDataTypeStr=Inherit: Same as first input
  Product4 : Product  InputSameDT=on  SaturateOnIntegerOverflow=on  OutDataTypeStr=Inherit: Same as first input
  S_ref : Gain  Gain=S_ref  SaturateOnIntegerOverflow=on  OutDataTypeStr=Inherit: Same as input  ParamDataTypeStr=Inherit: Same as input
  "S_ref " : Gain  Gain=S_ref  SaturateOnIntegerOverflow=on  OutDataTypeStr=Inherit: Same as input  ParamDataTypeStr=Inherit: Same as input
  S_ref X d_ref : Gain  Gain=S_ref * d_ref  SaturateOnIntegerOverflow=on  OutDataTypeStr=Inherit: Same as input  ParamDataTypeStr=Inherit: Same as input
  Fx : Outport  InitialOutput=[0]  VectorParamsAs1DForOutWhenUnconnected=off
  Fz : Outport  Port=2  InitialOutput=0  VectorParamsAs1DForOutWhenUnconnected=off
  " M" : Outport  Port=3  InitialOutput=0  VectorParamsAs1DForOutWhenUnconnected=off
  wires:
  Incidence/1(Cx_alpha) -> Cx_tot/1
  Fins/1(Cx_el) -> Cx_tot/2
  Incidence/2(Cz_alpha) -> Cz_tot/1
  Fins/2(Cz_el) -> Cz_tot/2
  Incidence/3(Cm_alpha) -> Cm_tot/1
  Fins/3(Cm_el) -> Cm_tot/2
  Body Rate/1 -> Cm_tot/3
  Alpha/1 -> Incidence/2(Alpha)
  Cx_tot/1 -> Product2/1
  Cz_tot/1 -> Product3/1
  Product2/1 -> S_ref/1
  S_ref/1 -> Fx/1
  Product3/1 -> "S_ref "/1
  "S_ref "/1 -> Fz/1
  Fin/1 -> Fins/1(Fin)
  S_ref X d_ref/1 -> " M"/1
  Product4/1 -> S_ref X d_ref/1
  Cm_tot/1 -> Product4/2
  Mach/1 -> Incidence/1(Mach)
  q/1 -> Body Rate/1
  Q/1 -> Product4/1, Product3/2, Product2/2

== system aero_guidance_train_2026/Airframe & Autopilot/Autopilot/Gain Scheduled Coefficients ==
  Alpha : Inport
  Mach : Inport  Port=2
  2-D Lookup Table : Lookup_n-D  BreakpointsForDimension1=M_sch  BreakpointsForDimension2=alpha_sch  Table=Ka  InternalRulePriority=Speed  RndMeth=Simplest
      settings: InputPortMap=u0,u1
  2-D Lookup Table1 : Lookup_n-D  BreakpointsForDimension1=M_sch  BreakpointsForDimension2=alpha_sch  Table=K  InternalRulePriority=Speed  RndMeth=Simplest
      settings: InputPortMap=u0,u1
  2-D Lookup Table2 : Lookup_n-D  BreakpointsForDimension1=M_sch  BreakpointsForDimension2=alpha_sch  Table=Ki  InternalRulePriority=Speed  RndMeth=Simplest
      settings: InputPortMap=u0,u1
  2-D Lookup Table3 : Lookup_n-D  BreakpointsForDimension1=M_sch  BreakpointsForDimension2=alpha_sch  Table=Kg  InternalRulePriority=Speed  RndMeth=Simplest
      settings: InputPortMap=u0,u1
  Abs : Abs
  "Kg " : Outport  InitialOutput=0  VectorParamsAs1DForOutWhenUnconnected=off
  "KI " : Outport  Port=2  InitialOutput=0  VectorParamsAs1DForOutWhenUnconnected=off
  "K " : Outport  Port=3  InitialOutput=0  VectorParamsAs1DForOutWhenUnconnected=off
  "Ka " : Outport  Port=4  InitialOutput=0  VectorParamsAs1DForOutWhenUnconnected=off
  wires:
  Alpha/1 -> Abs/1
  2-D Lookup Table/1 -> "Ka "/1
  2-D Lookup Table1/1 -> "K "/1
  2-D Lookup Table2/1 -> "KI "/1
  2-D Lookup Table3/1 -> "Kg "/1
  Mach/1 -> 2-D Lookup Table3/1, 2-D Lookup Table2/1, 2-D Lookup Table1/1, 2-D Lookup Table/1
  Abs/1 -> 2-D Lookup Table3/2, 2-D Lookup Table2/2, 2-D Lookup Table/2, 2-D Lookup Table1/2

== system aero_guidance_train_2026/Guidance/Fuze/Miss distance ==
  In1 : Inport
  Trigger : TriggerPort  VariantControl=(inherit)
  Display : Display
  wires:
  In1/1 -> Display/1  "Miss Distance"

== system aero_guidance_train_2026/Seeker//Tracker/Tracker and Sightline Rate Estimator/Estimator Filter ==
  Dish error : Inport
  q : Inport  Port=2
  Enable : EnablePort  StatesWhenEnabling=reset
  Integrator : Integrator  InitialConditionSource=external
  Sum : Sum  Inputs=|+-  InputSameDT=on  SaturateOnIntegerOverflow=on  OutDataTypeStr=Inherit: Same as first input
  Sum1 : Sum  Inputs=|+-  InputSameDT=on  SaturateOnIntegerOverflow=on  OutDataTypeStr=Inherit: Same as first input
  Sum5 : Sum  Inputs=|++  InputSameDT=on  SaturateOnIntegerOverflow=on  OutDataTypeStr=Inherit: Same as first input
  q_filt : Integrator
  wn_hom : Gain  Gain=wn_hom  SaturateOnIntegerOverflow=on  OutDataTypeStr=Inherit: Same as input  ParamDataTypeStr=Inherit: Same as input
  "wn_hom  " : Gain  Gain=wn_hom  SaturateOnIntegerOverflow=on  OutDataTypeStr=Inherit: Same as input  ParamDataTypeStr=Inherit: Same as input
  Sightline Rate : Outport  InitialOutput=0  VectorParamsAs1DForOutWhenUnconnected=off
  wires:
  Dish error/1 -> Sum/1, Integrator/2
  Sum/1 -> wn_hom/1
  Integrator/1 -> Sum/2
  Sum5/1 -> Sightline Rate/1
  wn_hom/1 -> Integrator/1, Sum5/1
  q/1 -> Sum1/1
  Sum1/1 -> "wn_hom  "/1
  "wn_hom  "/1 -> q_filt/1
  q_filt/1 -> Sum5/2, Sum1/2

== system aero_guidance_train_2026/Seeker//Tracker/Tracker and Sightline Rate Estimator/Switch to Closed Loop Tracking ==
  Dish Error : Inport
  Sigma_d : Inport  Port=2
  Gimbal : Inport  Port=3
  Guided Flight : Fcn  Expr=u(1)>1
  Sum5 : Sum  Inputs=-+  InputSameDT=on  SaturateOnIntegerOverflow=on  OutDataTypeStr=Inherit: Same as first input
  Switch2 : Switch  Threshold=0.5
  "Dish Error " : Outport  VectorParamsAs1DForOutWhenUnconnected=off
  wires:
  [Mode] -> Guided Flight/1
  Guided Flight/1 -> Switch2/2
  Sum5/1 -> Switch2/3
  Dish Error/1 -> Switch2/1
  Switch2/1 -> "Dish Error "/1
  Sigma_d/1 -> Sum5/2
  Gimbal/1 -> Sum5/1

== system aero_guidance_train_2026/Airframe & Autopilot/Aerodynamics & Equations of Motion/Aerodynamics/Fins ==
  Fin : Inport
  Cm : Gain  Gain=Cm_el  SaturateOnIntegerOverflow=on  OutDataTypeStr=Inherit: Same as input  ParamDataTypeStr=Inherit: Same as input
  Cx : Gain  Gain=0  SaturateOnIntegerOverflow=on  OutDataTypeStr=Inherit: Same as input  ParamDataTypeStr=Inherit: Same as input
  Cz : Gain  Gain=Cz_el  SaturateOnIntegerOverflow=on  OutDataTypeStr=Inherit: Same as input  ParamDataTypeStr=Inherit: Same as input
  Cx_el : Outport  InitialOutput=0  VectorParamsAs1DForOutWhenUnconnected=off
  Cz_el : Outport  Port=2  InitialOutput=0  VectorParamsAs1DForOutWhenUnconnected=off
  Cm_el : Outport  Port=3  InitialOutput=0  VectorParamsAs1DForOutWhenUnconnected=off
  wires:
  Fin/1 -> Cx/1, Cm/1, Cz/1
  Cx/1 -> Cx_el/1
  Cm/1 -> Cm_el/1
  Cz/1 -> Cz_el/1

== system aero_guidance_train_2026/Airframe & Autopilot/Aerodynamics & Equations of Motion/Aerodynamics/Incidence ==
  Mach : Inport
  Alpha : Inport  Port=2
  2-D Lookup Table : Lookup_n-D  BreakpointsForDimension1=alpha_vec  BreakpointsForDimension2=Mach_vec  Table=Cx_alpha  InternalRulePriority=Speed  RndMeth=Simplest
      settings: InputPortMap=u0,u1
  2-D Lookup Table1 : Lookup_n-D  BreakpointsForDimension1=alpha_vec  BreakpointsForDimension2=Mach_vec  Table=Cz_alpha  InternalRulePriority=Speed  RndMeth=Simplest
      settings: InputPortMap=u0,u1
  2-D Lookup Table2 : Lookup_n-D  BreakpointsForDimension1=alpha_vec  BreakpointsForDimension2=Mach_vec  Table=Cm_alpha  InternalRulePriority=Speed  RndMeth=Simplest
      settings: InputPortMap=u0,u1
  Cx_alpha : Outport  InitialOutput=0  VectorParamsAs1DForOutWhenUnconnected=off
  Cz_alpha : Outport  Port=2  InitialOutput=0  VectorParamsAs1DForOutWhenUnconnected=off
  Cm_alpha : Outport  Port=3  InitialOutput=0  VectorParamsAs1DForOutWhenUnconnected=off
  wires:
  Alpha/1 -> 2-D Lookup Table/1, 2-D Lookup Table2/1, 2-D Lookup Table1/1
  2-D Lookup Table/1 -> Cx_alpha/1
  2-D Lookup Table1/1 -> Cz_alpha/1
  Mach/1 -> 2-D Lookup Table2/2, 2-D Lookup Table1/2, 2-D Lookup Table/2
  2-D Lookup Table2/1 -> Cm_alpha/1

== matlab function aero_guidance_train_2026/Target Position/MATLAB Function1 ==
  data: range input; isDone output; t_now input; target_pos input; goal_pos input
function isDone = isDoneFunction(range, t_now, target_pos, goal_pos)
%#codegen
hit_distance = 10.0;
max_distance = 30000.0;
max_time     = 15.0;

X_goal = goal_pos(1);
Z_goal = goal_pos(2);
dist_to_goal = sqrt((target_pos(1) - X_goal)^2 + (target_pos(2) - Z_goal)^2);

is_hit      = (range <= hit_distance);
is_out      = (range >= max_distance);
is_time_out = (t_now >= max_time);
is_success  = dist_to_goal <= 200.0;

isDone = is_hit || is_out || is_time_out || is_success;
end

== stateflow chart aero_guidance_train_2026/Guidance/Guidance Processor (Updated @100Hz) ==
  settings: updateMethod=DISCRETE  sampleTime=0.01
  state Guidance [parallel]
    settings: executionOrder=1
    state Target_Search
      en: Mode=1;Sigma_d=0;incr=-100;Acquire_time=t;
      du: Sigma_d=Sigma_d+0.01*incr;
      Target_Search -> Target_Search [order 1] : [Sigma_d>30||Sigma_d<-30]  / incr=-incr;
    state Target_Lock
      en:Mode=2;Acquire_time=t;
    state Abort
      en:Detonate=1;
    state Radar_Guided
      en:Mode=3;
      ex:az_fix=az_dem;
    state Blind_Range
      en:Mode=4;
    (default) -> Target_Search : {az_fix=-9.81;}
    Radar_Guided -> Target_Search [order 1] : [Acquire==0]
    Target_Search -> Abort [order 2] : [t-Acquire_time>7]
        | / send(Timeout, Fuze);
    Target_Search -> Target_Lock [order 1] : [Acquire==1]
    Target_Lock -> Radar_Guided : [t-Acquire_time>0.2]
    Radar_Guided -> Blind_Range [order 2] : [Range<200]
  state Fuze [parallel]
    settings: executionOrder=2
    state Armed
      en:Fuze=1;
    state Inert
      en:Fuze = 0;
    Inert -> Armed [order 2] : [in(Guidance.Radar_Guided)&&Range<1000]
    (default) -> Inert
    Inert -> Armed [order 1] : Timeout
    Armed -> Inert : enter(Guidance.Target_Search)
  data: Range input double; Detonate output boolean; Fuze output boolean; Sigma_d output double; Mode output uint8; Acquire input boolean; Acquire_time local double; incr local double; az_dem input double; az_fix output double =-9.81
  data Sigma_d settings: description=Demanded Seeker Look Angle
  data Acquire settings: description=Seeker Acquisition Flag
  data incr settings: description=Seeker Search Rate
  events: Timeout local EITHER_EDGE_EVENT

== matlab function aero_guidance_train_2026/Target Position/targetMotionRL ==
  data: T_pos input; T_pos_next output; T_speed input; T_heading input; dt input; psi_dot_cmd input; T_vel output; T_heading_next output
function [T_pos_next, T_vel, T_heading_next] = targetMotionRL(T_pos, T_speed, T_heading, dt, psi_dot_cmd)
%#codegen
% 1) Heading update
T_heading_next = T_heading + psi_dot_cmd * dt;
T_heading_next = atan2(sin(T_heading_next), cos(T_heading_next));

% 2) Velocity update
T_vel = T_speed * [cos(T_heading_next); sin(T_heading_next)];

% 3) Position update
T_pos_next = [T_pos(1) + T_vel(1)*dt; T_pos(2) + T_vel(2)*dt];
end

== matlab function aero_guidance_train_2026/Target Position/RL Mode Manager ==
  data: range input; use_RL output; rl_started output; t_now input
function [use_RL, rl_started] = rlModeManager(range, t_now)
%#codegen

% 훈련 안정성을 위해 RL 모드를 항상 활성화 (스위칭 해제)
use_RL     = 1.0;
rl_started = 1.0;

end

== matlab function aero_guidance_train_2026/Target Position/MATLAB Function ==
  data: range input; reward output; rangeRate input; action_prev input; rl_started input; target_pos input; Goal_pos input
function reward = rewardFunction(range, rangeRate, action_prev, rl_started, target_pos, Goal_pos)
%#codegen

% RL이 시작되기 전(3500m 밖)에는 에이전트 학습 보상을 0으로 대기
if rl_started < 0.5
    reward = 0.0;
    return;
end

% --- 3500m 이내 진입 후 RL 작동 시 보상 로직 ---
X_goal = Goal_pos(1);
Z_goal = Goal_pos(2);
dist_to_goal = sqrt((target_pos(1) - X_goal)^2 + (target_pos(2) - Z_goal)^2);

if range <= 10.0
    reward = -200.0; % 격추 실패
    return;
elseif dist_to_goal <= 200.0
    reward = +300.0; % 목적지 도착 성공
    return;
end

% 타임스텝 보상
goal_reward   = -0.0001 * dist_to_goal; 
r_rate_reward = 2.0 * (rangeRate / 500.0); 
act_penalty   = 0.005 * (action_prev^2);

reward = 0.1 + goal_reward + r_rate_reward - act_penalty;

end
